simulink model "zwei_c"  (R2023a)
settings: Solver=VariableStepAuto  StartTime=0.0  StopTime=10.0  RelTol=1e-3
settings Model: Creator=alexa  LastModifiedBy=alexa

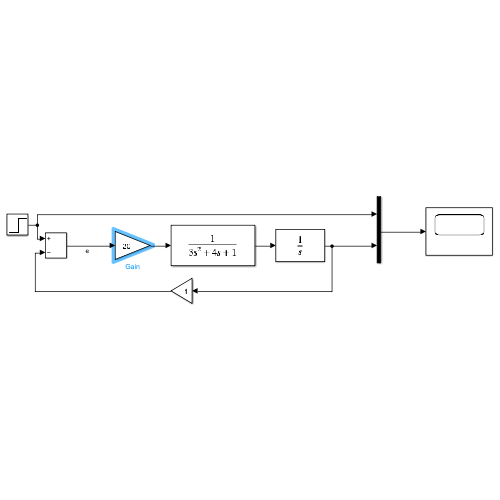
[thumbnail: Simulink's stored preview of the top-level diagram]
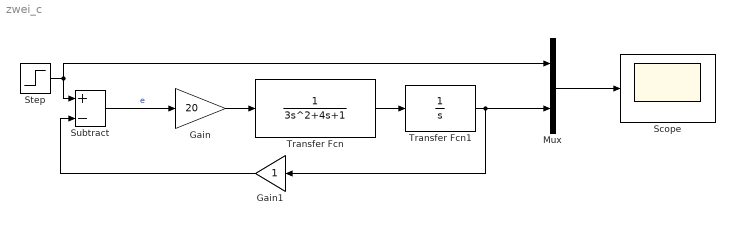
== system zwei_c ==
  Gain : Gain  Gain=20
  Gain1 : Gain
  Mux : Mux  Inputs=2
  Scope : Scope
  Step : Step  SampleTime=0
  Subtract : Sum  Inputs=+-
  Transfer Fcn : TransferFcn  Denominator=[3 4 1]
  Transfer Fcn1 : TransferFcn  Denominator=[1 0]
  wires:
  Step/1 -> Mux/1, Subtract/1
  Subtract/1 -> Gain/1  "e"
  Gain/1 -> Transfer Fcn/1
  Transfer Fcn/1 -> Transfer Fcn1/1
  Transfer Fcn1/1 -> Mux/2, Gain1/1
  Mux/1 -> Scope/1
  Gain1/1 -> Subtract/2
